simulink model "Lab2_2"  (R2012b)
settings: Solver=ode45  StartTime=0.0  StopTime=100  RelTol=1e-3
values from neighbouring files (symbols this model uses):
  tau = 2*pi/100/bw    [Lab2_2_open_loop_system.m]
libraries: simulink_extras x3, simulink x1
settings Model: Creator=Viktor  LastModifiedBy=Viktor

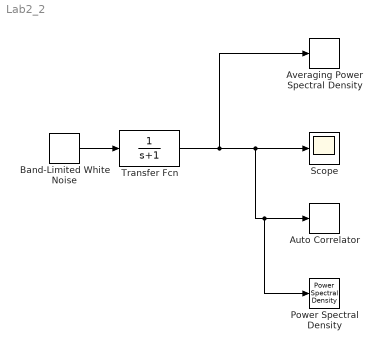
== system Lab2_2 ==
  Auto Correlator : simulink_extras/Additional Sinks/Auto Correlator  npts=100  HowOften=50  sampleT=tau
  Averaging Power Spectral Density : simulink_extras/Additional Sinks/Averaging Power Spectral Density  npts=128  fftpts=512  HowOften=64  sampleT=0.1
  Band-Limited White Noise : simulink/Sources/Band-Limited White Noise  Cov=1  Ts=tau  seed=[23341]
  Power Spectral Density : simulink_extras/Additional Sinks/Power Spectral Density  npts=128  fftpts=512  HowOften=64  sampleT=0.1
  Scope : Scope
      settings: SaveName=LinearSystemOutput  SampleInput=on  SampleTime=tau
  Transfer Fcn : TransferFcn  Denominator=[1 1]
  wires:
  Transfer Fcn/1 -> Averaging Power Spectral Density/1, Power Spectral Density/1, Auto Correlator/1, Scope/1
  Band-Limited White Noise/1 -> Transfer Fcn/1
